simulink model "ErrLmp"  (R2016b)
settings: Solver=VariableStepAuto  StartTime=0.0  StopTime=10.0  RelTol=1e-3
settings Model: Creator=jiakui  LastModifiedBy=jiakui

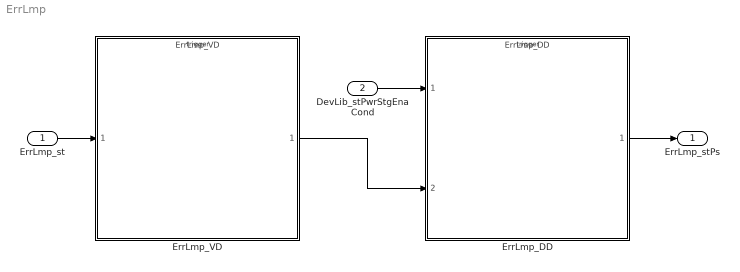
== system ErrLmp ==
  ErrLmp_st : Inport  Description=Error lamp status  OutMin=0  OutMax=1  OutDataTypeStr=boolean
  DevLib_stPwrStgEnaCond : Inport  Description=Control unit status relevant to power stage deactivation/error diagnosis  Port=2  OutMin=0  OutMax=65535  OutDataTypeStr=State_uint16
  ErrLmp_DD : ModelReference  ModelNameDialog=ErrLmp_DD  SimulationMode=Normal  ModelReferenceVersion=1.6  TriggerPortName=function  TriggerPortTriggerType=function-call  TriggerPortStatesWhenEnabling=held
  ErrLmp_VD : ModelReference  ModelNameDialog=ErrLmp_VD  SimulationMode=Normal  ModelReferenceVersion=1.3  TriggerPortName=function  TriggerPortTriggerType=function-call  TriggerPortStatesWhenEnabling=held
  ErrLmp_stPs : Outport  Description=Digital output to the actuator after diagnosis  OutMin=0  OutMax=1  OutDataTypeStr=boolean
  wires:
  ErrLmp_st/1 -> ErrLmp_VD/1
  ErrLmp_VD/1 -> ErrLmp_DD/2
  DevLib_stPwrStgEnaCond/1 -> ErrLmp_DD/1
  ErrLmp_DD/1 -> ErrLmp_stPs/1
